simulink model "AccGyrXSim"  (R2025b)
settings: Solver=VariableStepAuto  StartTime=0.0  StopTime=25  RelTol=1e-3
values from neighbouring files (symbols this model uses):
  Acc = [AccX.Data AccY.Data AccZ.Data]    [AccGyrX.m]
  Gyr = [GyrX.Data GyrY.Data GyrZ.Data]    [AccGyrX.m]
libraries: mspfiltlib x1
settings Model: Creator=HUB4RT  LastModifiedBy=HUB4RT

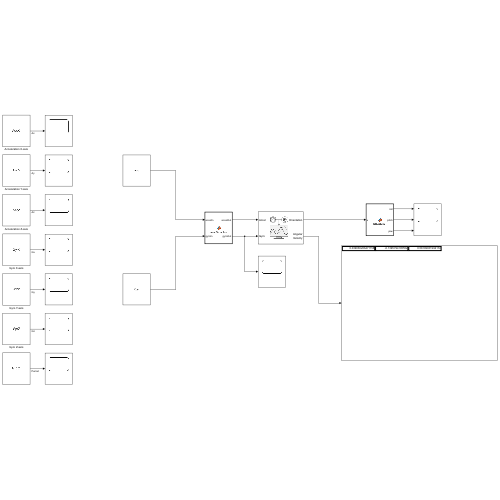
[thumbnail: Simulink's stored preview of the top-level diagram]
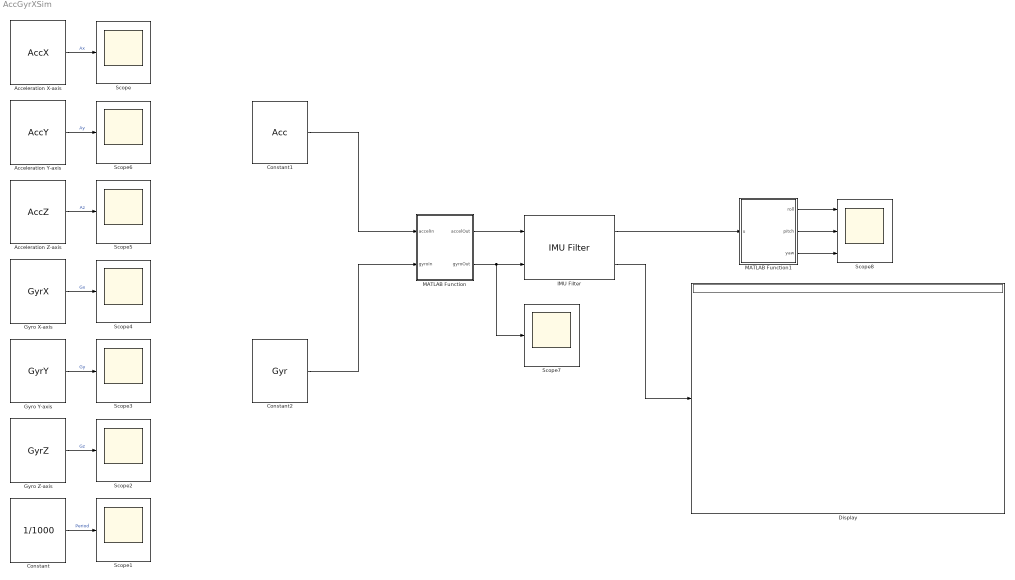
== system AccGyrXSim ==
  Acceleration X-axis : FromWorkspace  VariableName=AccX  SampleTime=0.001  OutputAfterFinalValue=Holding final value
  Acceleration Y-axis : FromWorkspace  VariableName=AccY  SampleTime=0.001  OutputAfterFinalValue=Holding final value
  Acceleration Z-axis : FromWorkspace  VariableName=AccZ  SampleTime=0.001  OutputAfterFinalValue=Holding final value
  Constant : Constant  Value=1/1000
  Constant1 : Constant  Value=Acc  SampleTime=0.02
  Constant2 : Constant  Value=Gyr  SampleTime=0.02
  Display : Display
      settings: Format=decimal (Stored Integer)
  Gyro X-axis : FromWorkspace  VariableName=GyrX  SampleTime=0.001  OutputAfterFinalValue=Holding final value
  Gyro Y-axis : FromWorkspace  VariableName=GyrY  SampleTime=0.001  OutputAfterFinalValue=Holding final value
  Gyro Z-axis : FromWorkspace  VariableName=GyrZ  SampleTime=0.001  OutputAfterFinalValue=Holding final value
  IMU Filter : mspfiltlib/IMU Filter  DispRefFrame=NED  OrientationFormat=quaternion  DecimationFactor=1  InitialProcessNoise=imufilter.defaultProcessNoise  AccelerometerNoise=0.0001924722  GyroscopeNoise=9.1385e-5  GyroscopeDriftNoise=3.0462e-13  LinearAccelerationNoise=0.0096236100000000012  LinearAccelerationDecayFactor=0.5  SimulateUsing=Interpreted execution
  MATLAB Function : MATLAB Function  TreatAsAtomicUnit=on
  MATLAB Function1 : MATLAB Function  TreatAsAtomicUnit=on
  Scope{,1..7} (8 alike) : Scope
      Scope settings: ActiveDisplayYMinimum=-1  ActiveDisplayYMaximum=1
      Scope2 settings: ActiveDisplayYMinimum=-1.1792788818076481  ActiveDisplayYMaximum=1.3732842431923526  DataLoggingVariableName=ScopeData2
      Scope3 settings: ActiveDisplayYMinimum=-1  ActiveDisplayYMaximum=1  DataLoggingVariableName=ScopeData3
      Scope4 settings: ActiveDisplayYMinimum=-1  ActiveDisplayYMaximum=1  DataLoggingVariableName=ScopeData4
      Scope5 settings: ActiveDisplayYMinimum=-1  ActiveDisplayYMaximum=1  DataLoggingVariableName=ScopeData5
      Scope6 settings: ActiveDisplayYMinimum=-1  ActiveDisplayYMaximum=1  DataLoggingVariableName=ScopeData6
      Scope7 settings: ActiveDisplayYMinimum=-4.1841086763342226  ActiveDisplayYMaximum=4.5433884541645053  DataLoggingVariableName=ScopeData7
  Scope8 : Scope  NumInputPorts=3
      settings: ActiveDisplayYMinimum=-140.38439066323915  ActiveDisplayYMaximum=95.4617178964652  DataLoggingVariableName=ScopeData8
  wires:
  Acceleration X-axis/1 -> Scope/1  "Ax"
  Constant/1 -> Scope1/1  "Period"
  Gyro Z-axis/1 -> Scope2/1  "Gz"
  Gyro Y-axis/1 -> Scope3/1  "Gy"
  Gyro X-axis/1 -> Scope4/1  "Gx"
  Acceleration Z-axis/1 -> Scope5/1  "Az"
  Acceleration Y-axis/1 -> Scope6/1  "Ay"
  Constant1/1 -> MATLAB Function/1(accelIn)
  Constant2/1 -> MATLAB Function/2(gyroIn)
  MATLAB Function/1(accelOut) -> IMU Filter/1
  MATLAB Function/2(gyroOut) -> Scope7/1, IMU Filter/2
  IMU Filter/2 -> Display/1
  IMU Filter/1 -> MATLAB Function1/1(u)
  MATLAB Function1/1(roll) -> Scope8/1
  MATLAB Function1/2(pitch) -> Scope8/2
  MATLAB Function1/3(yaw) -> Scope8/3

== matlab function AccGyrXSim/MATLAB Function ==
  data: accelIn input; accelOut output; gyroIn input; gyroOut output
function [accelOut,gyroOut] = readSamples(accelIn,gyroIn)

persistent selectSample;
if isempty(selectSample)
    selectSample = 0;
end
selectSample = selectSample + 1;

accelOut = accelIn(selectSample,:);
gyroOut = gyroIn(selectSample,:) * (2000.0/32768.0) * (pi/180.0);

== matlab function AccGyrXSim/MATLAB Function1 ==
  data: u input; roll output; pitch output; yaw output
function [roll, pitch, yaw] = hquat2eul(u)

q2 = quaternion(u(:,1), u(:,2), u(:,3), u(:,4));
y = eulerd(q2, "ZYX", "frame");

yaw = y(3);
pitch = y(2);
roll = y(1)-45;

roll  = mod(roll  + 180, 360) - 180;
pitch = mod(pitch + 180, 360) - 180;
yaw   = mod(yaw   + 180, 360) - 180;
